simulink model "modern_gnc"  (R2022b)
settings: Solver=VariableStepAuto  StartTime=0.0  StopTime=25  RelTol=1e-3
undefined symbols (not defined in the file): L
libraries: simulink x2, slpidlib x1, aerolibanimutils x1
settings Model: Creator=khush  LastModifiedBy=khush

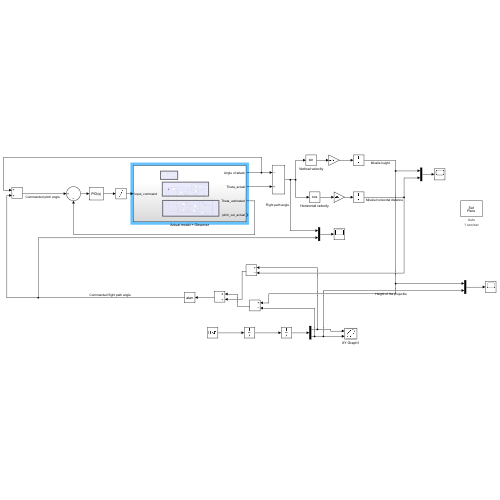
[thumbnail: Simulink's stored preview of the top-level diagram]
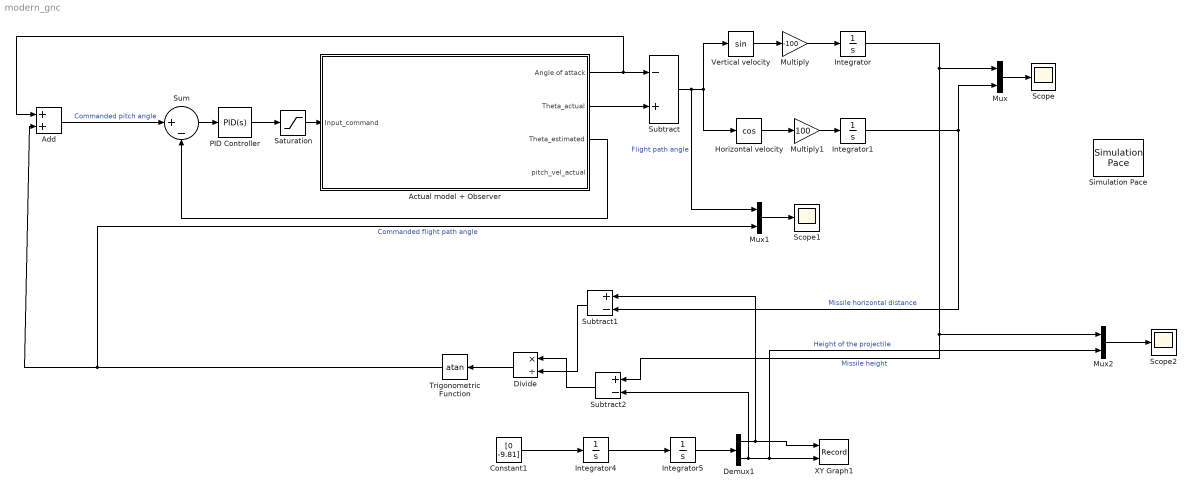
== system modern_gnc ==
  Actual model + Observer : Subsystem
  Add : Sum
  Constant1 : Constant  Value=[0 -9.81]
  Demux1 : Demux  Outputs=2
  Divide : Product  Inputs=*/
  Horizontal velocity : Trigonometry  Operator=cos
  Integrator : Integrator  InitialCondition=1000
  Integrator1 : Integrator
  Integrator4 : Integrator  InitialCondition=[100 100]
  Integrator5 : Integrator  InitialCondition=[0 0]
  Multiply : Gain  Gain=-100
  Multiply1 : Gain  Gain=100
  Mux : Mux  Inputs=2
  Mux1 : Mux  Inputs=2
  Mux2 : Mux  Inputs=2
  PID Controller : slpidlib/PID Controller  Controller=PID  Form=Parallel  TimeDomain=Continuous-time  UseExternalTs=off  SampleTime=-1  IntegratorMethod=Forward Euler  FilterMethod=Forward Euler  ControllerParametersSource=internal  P=-1  I=0.1  UseKiTs=off  D=.4  N=100  UseFilter=on  TunerSelectOption=Transfer Function Based (PID Tuner App)  InitialConditionSource=internal  InitialConditionForIntegrator=0  InitialConditionForFilter=0  DifferentiatorICPrevScaledInput=0  ExternalReset=none  TrackingMode=off  Kt=1  LimitOutput=off  SatLimitsSource=internal  UpperSaturationLimit=inf  LowerSaturationLimit=-inf  LinearizeAsGain=on  AntiWindupMode=none  Kb=1  LimitIntegrator=off  UpperIntegratorSaturationLimit=inf  LowerIntegratorSaturationLimit=-inf  POutMin=[]  POutMax=[]  IOutMin=[]  IOutMax=[]  DOutMin=[]  DOutMax=[]  NOutMin=[]  NOutMax=[]  SumOutMin=[]  SumOutMax=[]  SaturationOutMin=[]  SaturationOutMax=[]  PParamMin=[]  PParamMax=[]  IParamMin=[]  IParamMax=[]  DParamMin=[]  DParamMax=[]  NParamMin=[]  NParamMax=[]  KbParamMin=[]  KbParamMax=[]  KtParamMin=[]  KtParamMax=[]  KbOutMin=[]  KbOutMax=[]  KtOutMin=[]  KtOutMax=[]  IntegratorOutMin=[]  IntegratorOutMax=[]  FilterOutMin=[]  FilterOutMax=[]  SumI1OutMin=[]  SumI1OutMax=[]  SumI2OutMin=[]  SumI2OutMax=[]  SumI3OutMin=[]  SumI3OutMax=[]  SumI4OutMin=[]  SumI4OutMax=[]  SumDOutMin=[]  SumDOutMax=[]  DifferentiatorOutMin=[]  DifferentiatorOutMax=[]  FilterDiffOutCoefMin=[]  FilterDiffOutCoefMax=[]  ReciprocalOutMin=[]  ReciprocalOutMax=[]  SumDenOutMin=[]  SumDenOutMax=[]  SumNumOutMin=[]  SumNumOutMax=[]  DivideOutMin=[]  DivideOutMax=[]  UdiffTsProdOutMin=[]  UdiffTsProdOutMax=[]  NTsProdOutMin=[]  NTsProdOutMax=[]  UintegralTsProdOutMin=[]  UintegralTsProdOutMax=[]  UngainTsProdOutMin=[]  UngainTsProdOutMax=[]  ClampingZeroOutDataTypeStr=Inherit: Inherit via back propagation  ClampingZeroOutMin=[]  ClampingZeroOutMax=[]  FilterDenConstantOutDataTypeStr=Inherit: Inherit via back propagation  FilterDenConstantOutMin=[]  FilterDenConstantOutMax=[]  PCopyOutDataTypeStr=Inherit: Inherit via back propagation  PCopyOutMin=[]  PCopyOutMax=[]  NCopyOutDataTypeStr=Inherit: Inherit via back propagation  NCopyOutMin=[]  NCopyOutMax=[]  IntegratorContinuousStateAttributes=''  IntegratorStateMustResolveToSignalObject=off  IntegratorRTWStateStorageClass=Auto  FilterContinuousStateAttributes=''  FilterStateMustResolveToSignalObject=off  FilterRTWStateStorageClass=Auto  ParallelPVariant=InternalParameters  IdealPVariant=Disabled  IVariant=InternalParameters  DVariant=InternalParameters  IntegratorVariant=Continuous  SatVariant=Disabled  AWVariant=Passthrough  PCopyVariant=Disabled  TRVariant=Disabled  FdbkBlocksVariant=Forward  IdealPFdbkVariant=Disabled  SatFdbkVariant=Disabled  DerivativeFilterVariant=ContFilter  NVariant=InternalParameters  NCopyVariant=Disabled  FilterICVariant=InternalICsFilter  IntegratorICVariant=InternalICs  ExternalResetVariant=Disabled  TRSumVariant=Passthrough  SumFdbkVariant=Disabled  SumVariant=Sum_PID  TsampFilterVariant=InternalTs  TsampNgainVariant=Passthrough  TsampIntegralVariant=Passthrough  ExternalSaturationOutDataTypeStr=Inherit: Same as second input
  Saturation : Saturate  UpperLimit=1.5  LowerLimit=-1.5
  Scope : Scope
  Scope1 : Scope
  Scope2 : Scope
  Simulation Pace : aerolibanimutils/Simulation Pace  SimulationPace=1  SleepMode=Auto  OutputPaceError=off  SampleTime=1/30
  Subtract : Sum  Inputs=-+
  Subtract1 : Sum  Inputs=+-
  Subtract2 : Sum  Inputs=+-
  Sum : Sum  Inputs=|+-
  Trigonometric Function : Trigonometry  Operator=atan
  Vertical velocity : Trigonometry
  XY Graph1 : Record  FileSettingsInternal="{\"entries\":[{\"content\":{\"excelSettings\":{\"content\":{},\"type\":\"Streamout.ExcelSettings\"}},\"type\":\"Streamout.FileSettingStorage\",\"uuid\":\"d84a5269-7404-48e6-b449-5674176254c3\"}],\"packageUris\":[\"http://schema.mathworks.com/mf0/streamout_blocks/R2020a\"],\"version\":\"1.0\"}"  Layout=[1 1]  SignalsInternal="{\"entries\":[{\"content\":{\"signals\":[{\"content\":{\"blockPath\":[\"modern_gnc/XY Graph1\"],\"channel\":[],\"dimensions\":[1],\"domain\":\"modern_gnc/XY Graph1\",\"lineColor\":\"#a2142f\",\"plots\":[1],\"port\":1,\"sid\":[\"\"],\"signalID\":4428,\"signalName\":\"Demux1:1\"},\"type\":\"RecordBlkView.Signal\",\"uuid\":\"c3eb145d-45c6-4177-9713-50812e309298\"},{\"content\":{\"blockPath\":[\"modern_gnc/XY Graph1\"],\"channel\":[],\"dimensions\":[1],\"domain\":\"modern_gnc/XY Graph1\",\"lineColor\":\"#139fff\",\"plots\":[1],\"port\":2,\"sid\":[\"\"],\"signalID\":4432,\"signalName\":\"Demux1:2\"},\"type\":\"RecordBlkView.Signal\",\"uuid\":\"5104ca9c-935c-4818-8d8a-c9503e918009\"}]},\"type\":\"RecordBlkView.InputSignals\",\"uuid\":\"ae00ace9-5ecd-46bd-907b-941b64fb5323\"}],\"packageUris\":[\"http://schema.mathworks.com/mf0/streamout_blocks/R2020a\"],\"version\":\"1.0\"}"  VisualizationBindings="{\"xyplotplugin\":{\"info\":[{\"series\":[{\"bindingParametersList\":[{\"parameter\":\"X-Axis\",\"signalID\":4428,\"signalName\":\"Demux1:1\"},{\"parameter\":\"Y-Axis\",\"signalID\":4432,\"signalName\":\"Demux1:2\"}],\"seriesID\":36836}],\"subplotID\":1}]}}"  CompatibilityTag=XY
  wires:
  Sum/1 -> PID Controller/1
  Actual model + Observer/3(Theta_estimated) -> Sum/2
  Saturation/1 -> Actual model + Observer/1(Input_command)
  PID Controller/1 -> Saturation/1
  Actual model + Observer/1(Angle of attack) -> Add/1, Subtract/1
  Actual model + Observer/2(Theta_actual) -> Subtract/2
  Subtract/1 -> Mux1/1, Horizontal velocity/1, Vertical velocity/1  "Flight path angle"
  Vertical velocity/1 -> Multiply/1
  Horizontal velocity/1 -> Multiply1/1
  Multiply/1 -> Integrator/1
  Multiply1/1 -> Integrator1/1
  Integrator1/1 -> Subtract1/2, Mux/2  "Missile horizontal distance"
  Integrator/1 -> Mux2/1, Subtract2/1, Mux/1  "Missile height"
  Subtract2/1 -> Divide/1
  Subtract1/1 -> Divide/2
  Divide/1 -> Trigonometric Function/1
  Add/1 -> Sum/1  "Commanded pitch angle"
  Trigonometric Function/1 -> Mux1/2, Add/2  "Commanded flight path angle"
  Mux1/1 -> Scope1/1
  Mux/1 -> Scope/1
  Mux2/1 -> Scope2/1
  Integrator5/1 -> Demux1/1
  Constant1/1 -> Integrator4/1
  Demux1/2 -> Mux2/2, XY Graph1/2, Subtract2/2  "Height of the projectile"
  Demux1/1 -> Subtract1/1, XY Graph1/1
  Integrator4/1 -> Integrator5/1

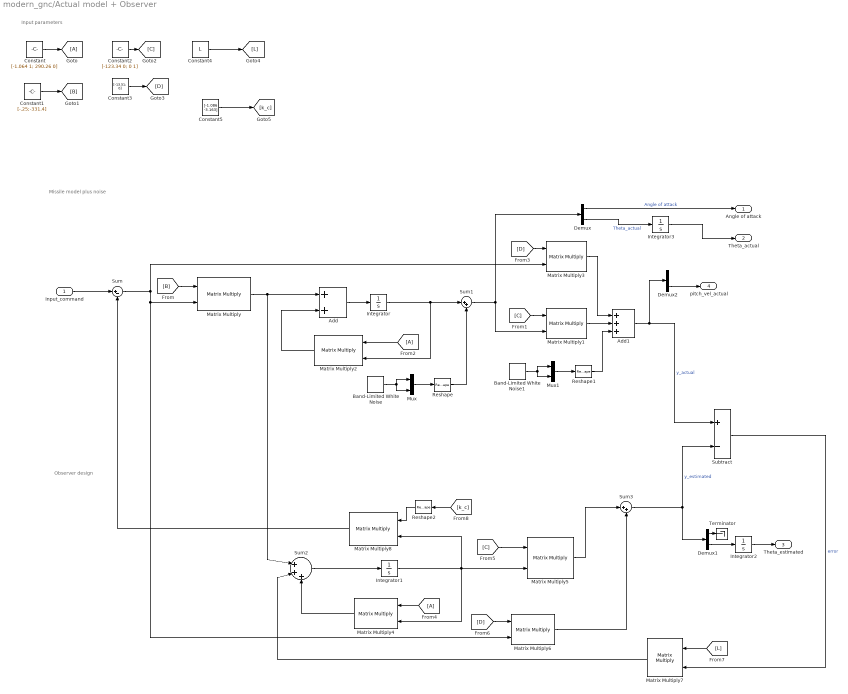
== system modern_gnc/Actual model + Observer ==
  note: Observer design
  note: Missile model plus noise
  note: Input parameters
  Input_command : Inport
  Add : Sum
  Add1 : Sum  Inputs=+++
  Band-Limited White Noise : simulink/Sources/Band-Limited White Noise  Cov=[0.00000001]  Ts=0.75  seed=[23341]
  Band-Limited White Noise1 : simulink/Sources/Band-Limited White Noise  Cov=[0.00000001]  Ts=0.25  seed=[23341]
  Constant : Constant  Value=[-1.064 1; 290.26 0]
  Constant1 : Constant  Value=[-.25;-331.4]
  Constant2 : Constant  Value=[-123.34 0; 0 1]
  Constant3 : Constant  Value=[-13.51; 0]
  Constant4 : Constant  Value=L
  Constant5 : Constant  Value=[-1.086 -3.163]
  Demux : Demux  Outputs=2
  Demux1 : Demux  Outputs=2
  Demux2 : Demux  Outputs=2
  From2 : From
  From4 : From
  Goto : Goto
  Integrator{,1..3} (4 alike) : Integrator
  Matrix Multiply{,1..8} (9 alike) : Product  Multiplication=Matrix(*)
  Mux : Mux  Inputs=2
  Mux1 : Mux  Inputs=2
  Reshape : Reshape  OutputDimensionality=Customize  OutputDimensions=[2,1]
  Reshape1 : Reshape  OutputDimensionality=Customize  OutputDimensions=[2,1]
  Reshape2 : Reshape  OutputDimensionality=Customize  OutputDimensions=[1,2]
  Subtract : Sum  Inputs=+-
  Sum : Sum  Inputs=|+-
  Sum1 : Sum  Inputs=|++
  Sum2 : Sum  Inputs=|+++
  Sum3 : Sum  Inputs=|++
  Terminator : Terminator
  Angle of attack : Outport
  Theta_actual : Outport  Port=2
  Theta_estimated : Outport  Port=3
  pitch_vel_actual : Outport  Port=4
  wires:
  Integrator/1 -> Matrix Multiply2/2, Sum1/1
  Matrix Multiply8/1 -> Sum/2
  [k_c] -> Reshape2/1
  [D] -> Matrix Multiply3/1
  Input_command/1 -> Sum/1
  Reshape2/1 -> Matrix Multiply8/1
  Mux/1 -> Reshape/1
  Constant3/1 -> [D]
  Sum/1 -> Matrix Multiply6/2, Matrix Multiply/2, Matrix Multiply3/2
  [C] -> Matrix Multiply1/1
  Add/1 -> Integrator/1
  Constant4/1 -> [L]
  Reshape/1 -> Sum1/2
  Band-Limited White Noise/1 -> Mux/2, Mux/1
  Band-Limited White Noise1/1 -> Mux1/1, Mux1/2
  Demux1/1 -> Terminator/1
  Reshape1/1 -> Add1/3
  Matrix Multiply6/1 -> Sum3/2
  From4/1 -> Matrix Multiply4/1
  Matrix Multiply4/1 -> Sum2/3
  Sum3/1 -> Demux1/1, Subtract/2  "y_estimated"
  Add1/1 -> Demux2/1, Subtract/1  "y_actual"
  Mux1/1 -> Reshape1/1
  [B] -> Matrix Multiply/1
  Integrator1/1 -> Matrix Multiply8/2, Matrix Multiply5/2, Matrix Multiply4/2
  Demux/1 -> Angle of attack/1  "Angle of attack"
  [D] -> Matrix Multiply6/1
  Constant2/1 -> [C]
  Sum1/1 -> Matrix Multiply1/2, Demux/1
  Matrix Multiply2/1 -> Add/2
  Matrix Multiply3/1 -> Add1/1
  Matrix Multiply/1 -> Sum2/1, Add/1
  Matrix Multiply5/1 -> Sum3/1
  Constant/1 -> Goto/1
  Matrix Multiply1/1 -> Add1/2
  Subtract/1 -> Matrix Multiply7/2  "error"
  Constant1/1 -> [B]
  From2/1 -> Matrix Multiply2/1
  Matrix Multiply7/1 -> Sum2/2
  [C] -> Matrix Multiply5/1
  Sum2/1 -> Integrator1/1
  [L] -> Matrix Multiply7/1
  Constant5/1 -> [k_c]
  Demux1/2 -> Integrator2/1
  Integrator2/1 -> Theta_estimated/1
  Demux/2 -> Integrator3/1  "Theta_actual"
  Integrator3/1 -> Theta_actual/1
  Demux2/2 -> pitch_vel_actual/1
